simulink model "cantileverdamped"  (Simulink 9.2)
settings: Solver=ode45  StartTime=0.0  StopTime=200  MaxStep=0.001  RelTol=1e-3  EnableMultiTasking=on
settings Model: Creator=acer  LastModifiedBy=ASUS
settings OptimizationCC: ExpressionDepthLimit=2147483647  InitFltsAndDblsToZero=on
settings DebuggingCC: SaveWithParameterizedLinksMsg=none  SolverPrmCheckMsg=warning
settings SFSimCC: SimUseLocalCustomCode=on  SimParseCustomCode=off
settings RTWCC: RTWUseLocalCustomCode=on
settings GRTTargetCC: TargetFcnLib=ansi_tfl_tmw.mat  GeneratePreprocessorConditionals=Use local settings
settings ConfigComp: CovExternalEMLEnable=on

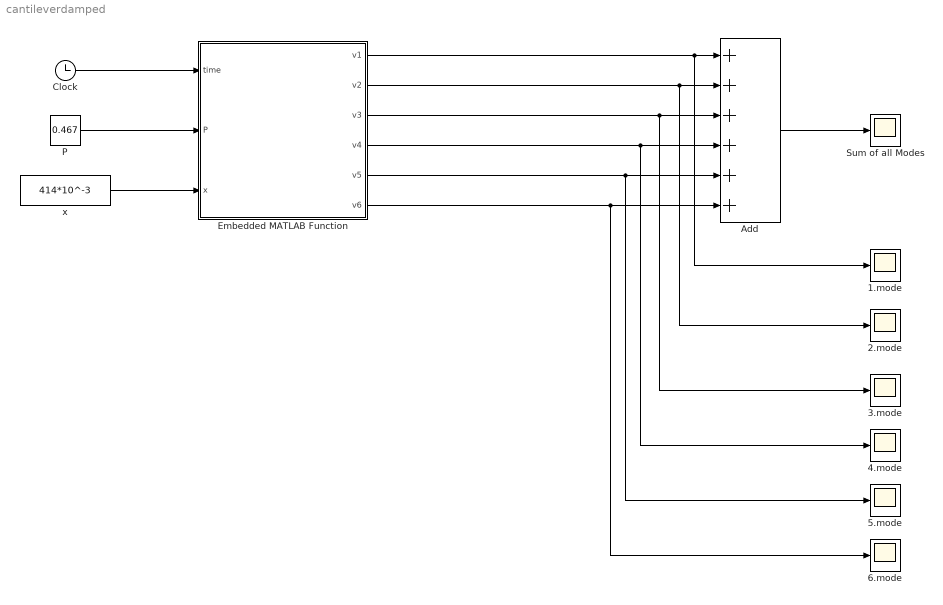
== system cantileverdamped ==
  1.mode : Scope
  2.mode : Scope
  3.mode : Scope
  4.mode : Scope
  "5.mode " : Scope
  6.mode : Scope
  Add : Sum  Inputs=++++++
  Clock : Clock
  Embedded MATLAB Function : MATLAB Function  TreatAsAtomicUnit=on
  P : Constant  Value=0.467
  Sum of all Modes : Scope
  x : Constant  Value=414*10^-3
  wires:
  x/1 -> Embedded MATLAB Function/3(x)
  Embedded MATLAB Function/4(v4) -> Add/4, 4.mode/1
  Embedded MATLAB Function/5(v5) -> Add/5, "5.mode "/1
  Add/1 -> Sum of all Modes/1
  P/1 -> Embedded MATLAB Function/2(P)
  Clock/1 -> Embedded MATLAB Function/1(time)
  Embedded MATLAB Function/1(v1) -> Add/1, 1.mode/1
  Embedded MATLAB Function/2(v2) -> Add/2, 2.mode/1
  Embedded MATLAB Function/3(v3) -> Add/3, 3.mode/1
  Embedded MATLAB Function/6(v6) -> Add/6, 6.mode/1

== matlab function Embedded MATLAB Function ==
  data: time input double; v1 output double; P input double; x input double; v2 output double; v3 output double; v4 output double; v5 output double; v6 output double
function [v1,v2,v3,v4,v5,v6] = fcn(time,P,x)

L=414*10^-3 ; %m 
w=14.88*10^-3 ; %m 
t=1*10^-3 ; %m
A=w*t ; %m^2
ro=5186.5 ; %kg/m^2 (Linear mass density)
E=70*10^9 ; %N/m^2
I=((w*(t^3))/12) ; 
lamda=A*ro ; 
ksi=1.42*10^-3 ;

k1=1.875104069/L ;
k2=4.694091133/L ;
k3=7.854757438/L ;
k4=10.99554073/L ; 
k5=14.13716839/L ;
k6=17.27875953/L ;

w1=(sqrt((((k1)^4)*E*I)/(lamda))) ;
w2=(sqrt((((k2)^4)*E*I)/(lamda))) ;
w3=(sqrt((((k3)^4)*E*I)/(lamda))) ;
w4=(sqrt((((k4)^4)*E*I)/(lamda))) ; 
w5=(sqrt((((k5)^4)*E*I)/(lamda))) ;
w6=(sqrt((((k6)^4)*E*I)/(lamda))) ;



wd1=w1*(sqrt(1-(ksi^2))) ;
wd2=w2*(sqrt(1-(ksi^2))) ;
wd3=w3*(sqrt(1-(ksi^2))) ;
wd4=w4*(sqrt(1-(ksi^2))) ;
wd5=w5*(sqrt(1-(ksi^2))) ;
wd6=w6*(sqrt(1-(ksi^2))) ;


A1=((-4*P.*L)./(E*I*lamda*((k1)^4)*((sin(k1*L)*exp(k1*L))+exp(2*k1*L)-1))).*((3*sin(k1*L)*(exp(2*k1*L)+1))-(2*((k1*L)^3)*exp(k1*L))+(cos(k1*L)*(3-(((k1*L)^3)*(exp(2*k1*L)+1))-(3*exp(2*k1*L))))) ;
A2=((-4*P.*L)./(E*I*lamda*((k2)^4)*((sin(k2*L)*exp(k2*L))+exp(2*k2*L)-1))).*((3*sin(k2*L)*(exp(2*k2*L)+1))-(2*((k2*L)^3)*exp(k2*L))+(cos(k2*L)*(3-(((k2*L)^3)*(exp(2*k2*L)+1))-(3*exp(2*k2*L))))) ;
A3=((-4*P.*L)./(E*I*lamda*((k3)^4)*((sin(k3*L)*exp(k3*L))+exp(2*k3*L)-1))).*((3*sin(k3*L)*(exp(2*k3*L)+1))-(2*((k3*L)^3)*exp(k3*L))+(cos(k3*L)*(3-(((k3*L)^3)*(exp(2*k3*L)+1))-(3*exp(2*k3*L))))) ;
A4=((-4*P.*L)./(E*I*lamda*((k4)^4)*((sin(k4*L)*exp(k4*L))+exp(2*k4*L)-1))).*((3*sin(k4*L)*(exp(2*k4*L)+1))-(2*((k4*L)^3)*exp(k4*L))+(cos(k4*L)*(3-(((k4*L)^3)*(exp(2*k4*L)+1))-(3*exp(2*k4*L))))) ;
A5=((-4*P.*L)./(E*I*lamda*((k5)^4)*((sin(k5*L)*exp(k5*L))+exp(2*k5*L)-1))).*((3*sin(k5*L)*(exp(2*k5*L)+1))-(2*((k5*L)^3)*exp(k5*L))+(cos(k5*L)*(3-(((k5*L)^3)*(exp(2*k5*L)+1))-(3*exp(2*k5*L))))) ;
A6=((-4*P.*L)./(E*I*lamda*((k6)^4)*((sin(k6*L)*exp(k6*L))+exp(2*k6*L)-1))).*((3*sin(k6*L)*(exp(2*k6*L)+1))-(2*((k6*L)^3)*exp(k6*L))+(cos(k6*L)*(3-(((k6*L)^3)*(exp(2*k6*L)+1))-(3*exp(2*k6*L))))) ;

beta1=k1 ;
beta2=k2 ;
beta3=k3 ;
beta4=k4 ;
beta5=k5 ;
beta6=k6 ;

gama1=(sinh(beta1*L)-sin(beta1*L))/(cosh(beta1*L)+cos(beta1*L)) ;
gama2=(sinh(beta2*L)-sin(beta2*L))/(cosh(beta2*L)+cos(beta2*L)) ;
gama3=(sinh(beta3*L)-sin(beta3*L))/(cosh(beta3*L)+cos(beta3*L)) ;
gama4=(sinh(beta4*L)-sin(beta4*L))/(cosh(beta4*L)+cos(beta4*L)) ;
gama5=(sinh(beta5*L)-sin(beta5*L))/(cosh(beta5*L)+cos(beta5*L)) ;
gama6=(sinh(beta6*L)-sin(beta6*L))/(cosh(beta6*L)+cos(beta6*L)) ;

C2=1;

X1=C2*(cosh((k1*L).*x./L)-cos((k1*L).*x./L)-gama1.*(sinh((k1*L).*x./L)-sin((k1*L).*x./L))) ;
X2=C2*(cosh((k2*L).*x./L)-cos((k2*L).*x./L)-gama2.*(sinh((k2*L).*x./L)-sin((k2*L).*x./L))) ;
X3=C2*(cosh((k3*L).*x./L)-cos((k3*L).*x./L)-gama3.*(sinh((k3*L).*x./L)-sin((k3*L).*x./L))) ;
X4=C2*(cosh((k4*L).*x./L)-cos((k4*L).*x./L)-gama4.*(sinh((k4*L).*x./L)-sin((k4*L).*x./L))) ;
X5=C2*(cosh((k5*L).*x./L)-cos((k5*L).*x./L)-gama5.*(sinh((k5*L).*x./L)-sin((k5*L).*x./L))) ;
X6=C2*(cosh((k6*L).*x./L)-cos((k6*L).*x./L)-gama6.*(sinh((k6*L).*x./L)-sin((k6*L).*x./L))) ;


q1=(exp(-ksi*w1.*time)).*cos(wd1*time);
q2=(exp(-ksi*w2.*time)).*cos(wd2*time);
q3=(exp(-ksi*w3.*time)).*cos(wd3*time);
q4=(exp(-ksi*w4.*time)).*cos(wd4*time);
q5=(exp(-ksi*w5.*time)).*cos(wd5*time);
q6=(exp(-ksi*w6.*time)).*cos(wd6*time);


v1=X1.*A1.*q1 ;
v2=X2.*A2.*q2 ;
v3=X3.*A3.*q3 ; 
v4=X4.*A4.*q4 ;
v5=X5.*A5.*q5 ;
v6=X6.*A6.*q6 ;
